simulink model "pvpanelPaper_3"  (R2020a)
settings: Solver=VariableStepAuto  StartTime=0.0  StopTime=10.0  RelTol=1e-3
settings Model: Creator=shrad  LastModifiedBy=shrad

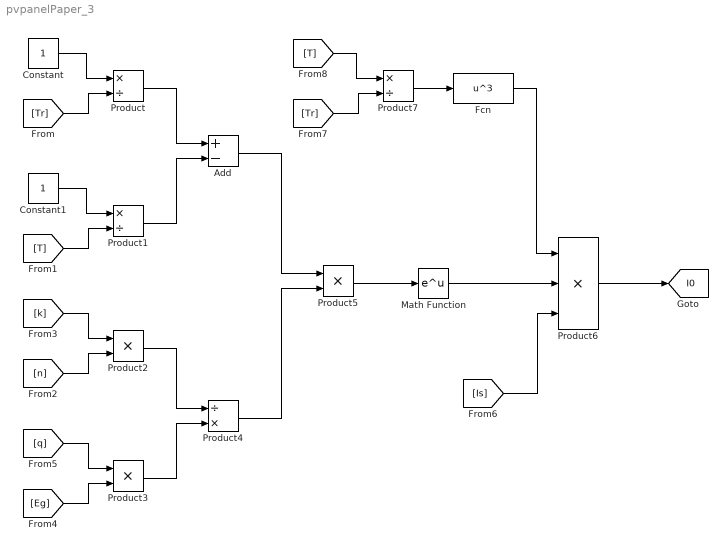
== system pvpanelPaper_3 ==
  Add : Sum  Inputs=+-
  Constant : Constant
  Constant1 : Constant
  Fcn : Fcn  Expr=u^3
  Math Function : Math  SaturateOnIntegerOverflow=on
  Product : Product  Inputs=*/
  Product1 : Product  Inputs=*/
  Product2 : Product  Inputs=**
  Product3 : Product  Inputs=**
  Product4 : Product  Inputs=/*
  Product5 : Product  Inputs=**
  Product6 : Product  Inputs=***
  Product7 : Product  Inputs=*/
  tag scope: I0=global
  wires:
  Constant/1 -> Product/1
  [Tr] -> Product/2
  [T] -> Product1/2
  Constant1/1 -> Product1/1
  [n] -> Product2/2
  [k] -> Product2/1
  [q] -> Product3/1
  [Eg] -> Product3/2
  Product2/1 -> Product4/1
  Product3/1 -> Product4/2
  Product/1 -> Add/1
  Product1/1 -> Add/2
  Add/1 -> Product5/1
  Product4/1 -> Product5/2
  Product5/1 -> Math Function/1
  Math Function/1 -> Product6/2
  [Is] -> Product6/3
  [Tr] -> Product7/2
  [T] -> Product7/1
  Product7/1 -> Fcn/1
  Fcn/1 -> Product6/1
  Product6/1 -> [I0]
